simulink model "multiplexer"  (R2023b)
settings: Solver=VariableStepAuto  StartTime=0.0  StopTime=10.0  RelTol=1e-3
settings Model: Creator=1234  LastModifiedBy=1234

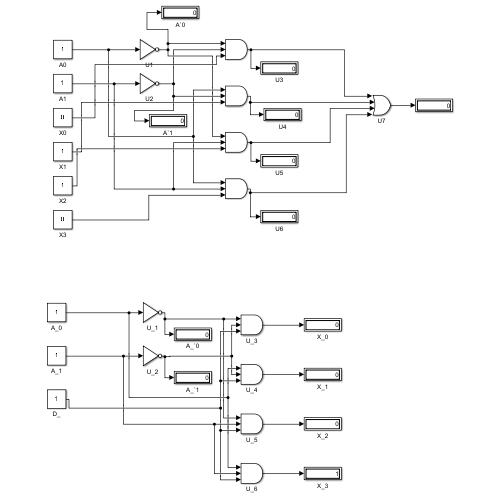
[thumbnail: Simulink's stored preview of the top-level diagram]
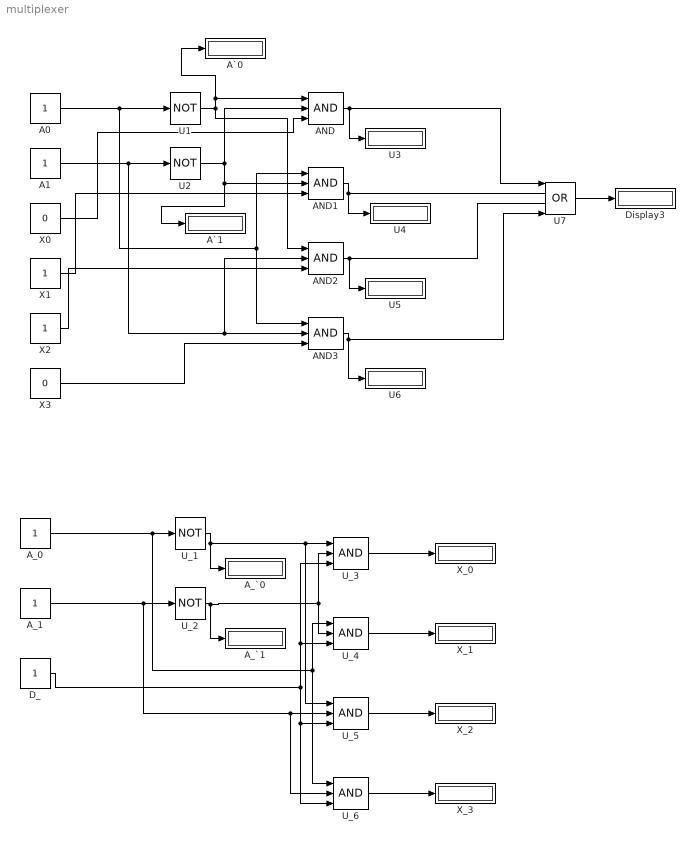
== system multiplexer ==
  A0 : Constant
  A1 : Constant
  AND{,1..3} (4 alike) : Logic  Inputs=3  IconShape=distinctive  AllPortsSameDT=off  OutDataTypeStr=boolean
  A_0 : Constant
  A_1 : Constant
  A_`0 : Display
  A_`1 : Display
  A`0 : Display
  A`1 : Display
  D_ : Constant
  Display3 : Display
  U1 : Logic  Operator=NOT  IconShape=distinctive  AllPortsSameDT=off  OutDataTypeStr=boolean
  U2 : Logic  Operator=NOT  IconShape=distinctive  AllPortsSameDT=off  OutDataTypeStr=boolean
  U{3..6} (4 alike) : Display
  U7 : Logic  Operator=OR  Inputs=4  IconShape=distinctive  AllPortsSameDT=off  OutDataTypeStr=boolean
  U_1 : Logic  Operator=NOT  IconShape=distinctive  AllPortsSameDT=off  OutDataTypeStr=boolean
  U_2 : Logic  Operator=NOT  IconShape=distinctive  AllPortsSameDT=off  OutDataTypeStr=boolean
  U_{3..6} (4 alike) : Logic  Inputs=3  IconShape=distinctive  AllPortsSameDT=off  OutDataTypeStr=boolean
  X0 : Constant  Value=0
  X1 : Constant
  X2 : Constant
  X3 : Constant  Value=0
  X_{0..3} (4 alike) : Display
  wires:
  A0/1 -> AND3/1, AND1/1, U1/1
  A1/1 -> AND2/2, AND3/2, U2/1
  U7/1 -> Display3/1
  AND/1 -> U3/1, U7/1
  AND1/1 -> U4/1, U7/2
  AND2/1 -> U5/1, U7/3
  AND3/1 -> U6/1, U7/4
  U1/1 -> AND/1, A`0/1, AND2/1
  U2/1 -> AND1/2, A`1/1, AND/2
  X0/1 -> AND/3
  X1/1 -> AND1/3
  X2/1 -> AND2/3
  X3/1 -> AND3/3
  U_3/1 -> X_0/1
  U_4/1 -> X_1/1
  U_6/1 -> X_3/1
  U_5/1 -> X_2/1
  A_0/1 -> U_4/1, U_6/1, U_1/1
  A_1/1 -> U_6/2, U_5/2, U_2/1
  U_1/1 -> U_5/1, U_3/1, A_`0/1
  U_2/1 -> U_3/2, U_4/2, A_`1/1
  D_/1 -> U_5/3, U_6/3, U_4/3, U_3/3
